simulink model "GFL_inverter2019a"  (R2019a)
settings: Solver=ode4  StartTime=0.0  StopTime=2  FixedStep=1e-6  RelTol=1e-3
values from neighbouring files (symbols this model uses):
  An1 = 0.01*funn    (= 0.3)    [dq_saopin_for_GFL_inverter.m]
  An2 = 0.03*funn    (= 0.9)    [dq_saopin_for_GFL_inverter.m]
  An3 = 0.05*funn    (= 1.5)    [dq_saopin_for_GFL_inverter.m]
  An4 = 0.07*funn    (= 2.1)    [dq_saopin_for_GFL_inverter.m]
  An5 = 0.09*funn    (= 2.7)    [dq_saopin_for_GFL_inverter.m]
  Ap1 = 0.01*funp    (= 0)    [dq_saopin_for_GFL_inverter.m]
  Ap2 = 0.03*funp    (= 0)    [dq_saopin_for_GFL_inverter.m]
  Ap3 = 0.05*funp    (= 0)    [dq_saopin_for_GFL_inverter.m]
  Ap4 = 0.07*funp    (= 0)    [dq_saopin_for_GFL_inverter.m]
  Ap5 = 0.09*funp    (= 0)    [dq_saopin_for_GFL_inverter.m]
  hp1 = hp0(n0)    [dq_saopin_for_GFL_inverter.m]
  hp2 = hp0(n0+hpn)    [dq_saopin_for_GFL_inverter.m]
  hp3 = hp0(n0+2*hpn)    [dq_saopin_for_GFL_inverter.m]
  hp4 = hp0(n0+3*hpn)    [dq_saopin_for_GFL_inverter.m]
  hp5 = hp0(n0+4*hpn)    [dq_saopin_for_GFL_inverter.m]
libraries: powerlib x27, powerlib_meascontrol x3, simulink x1
settings Model: Creator=18829  LastModifiedBy=wz
settings DataIOCC: ReturnWorkspaceOutputs=off
settings DebuggingCC: ArithmeticOperatorsInVariantConditions=warning
settings SFSimCC: SimUseLocalCustomCode=off
settings RTWCC: RTWUseLocalCustomCode=off
settings CodeAppCC: StateflowObjectComments=on
settings ConfigComp: CovBoundaryAbsTol=1.0e-5
settings SimscapeCC: SimscapeNormalizeSystem=off

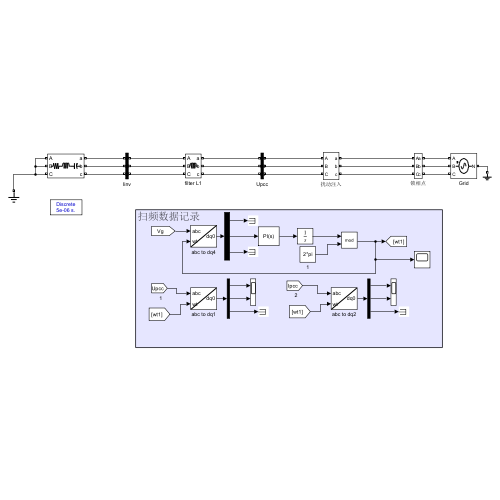
[thumbnail: Simulink's stored preview of the top-level diagram]
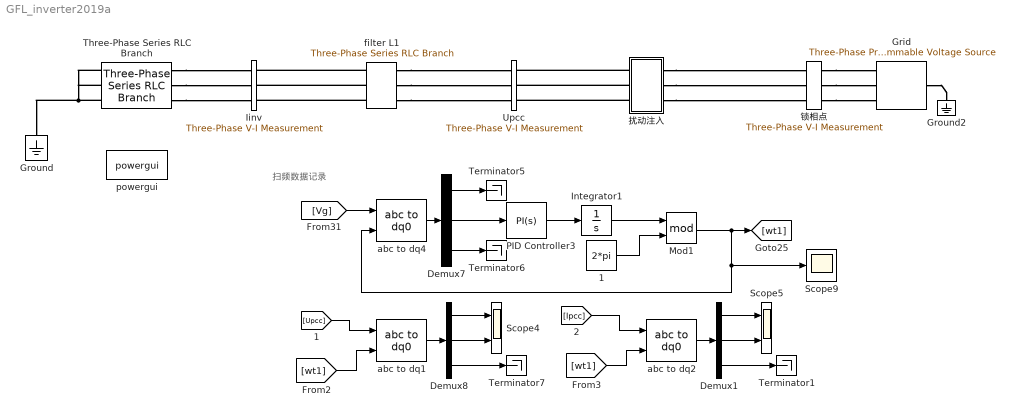
== system GFL_inverter2019a ==
  note: 扫频数据记录
  1 : Constant  Value=2*pi
  Demux1 : Demux  Outputs=3
  Demux7 : Demux  Outputs=3
  Demux8 : Demux  Outputs=3
  Grid : powerlib/Electrical Sources/Three-Phase Programmable Voltage Source  PositiveSequence=[380 0 50]  VariationEntity=None  VariationType=Table of time-amplitude pairs  VariationTypeAlt=Step  VariationStep=-3  VariationRate=10  VariationMagnitude=0.1  VariationFrequency=2  VariationTiming=[0.5 1.5]  VariationPhaseA=off  Amplitudes=[1 0.5 1]  TimeValues=[0 0.5 1]  HarmonicGeneration=off  HarmonicA=[7 0.1 0 0]  HarmonicB=[7 0.1 0 2]  Timing="[0.5  1]"  BusType=swing  Pref=0  Qref=0  Qmin=-inf  Qmax=inf
  Ground : powerlib/Elements/Ground  LConnTagsString=a
  Ground2 : powerlib/Elements/Ground  LConnTagsString=a
  Iinv : powerlib/Measurements/Three-Phase V-I Measurement  VoltageMeasurement=no  SetLabelV=off  LabelV=Uinv  Vpu=off  VpuLL=off  CurrentMeasurement=no  SetLabelI=off  LabelI=Iinv  Ipu=off  Pbase=100e6  Vbase=500e3  OutputType=Complex  PhasorSimulation=off  PSBequivalent=0
  Integrator1 : Integrator
  Mod1 : Math  Operator=mod  SaturateOnIntegerOverflow=on
  PID Controller3 : simulink/Continuous/PID Controller  Controller=PI  Form=Parallel  TimeDomain=Continuous-time  SampleTime=-1  IntegratorMethod=Forward Euler  ControllerParametersSource=internal  P=0.6935  I=74.885  D=0  N=100  UseFilter=on  TunerSelectOption=Transfer Function Based (PID Tuner App)  InitialConditionSource=internal  InitialConditionForIntegrator=100*pi  InitialConditionForFilter=0  DifferentiatorICPrevScaledInput=0  ExternalReset=none  TrackingMode=off  Kt=1  LimitOutput=off  UpperSaturationLimit=inf  LowerSaturationLimit=-inf  LinearizeAsGain=on  AntiWindupMode=none  Kb=1  POutMin=[]  POutMax=[]  IOutMin=[]  IOutMax=[]  DOutMin=[]  DOutMax=[]  NOutMin=[]  NOutMax=[]  SumOutMin=[]  SumOutMax=[]  SaturationOutMin=[]  SaturationOutMax=[]  PParamMin=[]  PParamMax=[]  IParamMin=[]  IParamMax=[]  DParamMin=[]  DParamMax=[]  NParamMin=[]  NParamMax=[]  KbParamMin=[]  KbParamMax=[]  KtParamMin=[]  KtParamMax=[]  KbOutMin=[]  KbOutMax=[]  KtOutMin=[]  KtOutMax=[]  IntegratorOutMin=[]  IntegratorOutMax=[]  FilterOutMin=[]  FilterOutMax=[]  SumI1OutMin=[]  SumI1OutMax=[]  SumI2OutMin=[]  SumI2OutMax=[]  SumI3OutMin=[]  SumI3OutMax=[]  SumI4OutMin=[]  SumI4OutMax=[]  SumDOutMin=[]  SumDOutMax=[]  DifferentiatorOutMin=[]  DifferentiatorOutMax=[]  FilterDiffOutCoefMin=[]  FilterDiffOutCoefMax=[]  ReciprocalOutMin=[]  ReciprocalOutMax=[]  SumDenOutMin=[]  SumDenOutMax=[]  SumNumOutMin=[]  SumNumOutMax=[]  DivideOutMin=[]  DivideOutMax=[]  IntegratorContinuousStateAttributes=''  IntegratorStateMustResolveToSignalObject=off  IntegratorRTWStateStorageClass=Auto  FilterContinuousStateAttributes=''  FilterStateMustResolveToSignalObject=off  FilterRTWStateStorageClass=Auto  ParallelPVariant=InternalParameters  IdealPVariant=Disabled  IVariant=InternalParameters  DVariant=Disabled  IntegratorVariant=Continuous  SatVariant=Disabled  AWVariant=Passthrough  PCopyVariant=Disabled  TRVariant=Disabled  FdbkBlocksVariant=Forward  IdealPFdbkVariant=Disabled  SatFdbkVariant=Disabled  DerivativeFilterVariant=Disabled  NVariant=Disabled  NCopyVariant=Disabled_SignalSpec  FilterICVariant=Disabled  IntegratorICVariant=InternalICs  ExternalResetVariant=Disabled  TRSumVariant=Passthrough  SumFdbkVariant=Disabled  SumVariant=Sum_PI
  Scope4 : Scope  NumInputPorts=2
  Scope5 : Scope  NumInputPorts=2
  Scope9 : Scope
  Terminator{1,5..7} (4 alike) : Terminator
  Three-Phase Series RLC Branch : powerlib/Elements/Three-Phase Series RLC Branch  LConnTagsString=A|B|C  RConnTagsString=A|B|C  BranchType=RLC  Resistance=1  Inductance=1e-3  Capacitance=0  Measurements=None
  Upcc : powerlib/Measurements/Three-Phase V-I Measurement  VoltageMeasurement=phase-to-ground  SetLabelV=on  LabelV=Upcc  Vpu=off  VpuLL=off  CurrentMeasurement=yes  SetLabelI=on  LabelI=Ipcc  Ipu=off  Pbase=100e6  Vbase=500e3  OutputType=Complex  PhasorSimulation=off  PSBequivalent=0
  abc to dq1 : powerlib_meascontrol/Transformations/abc to dq0  Alignment=90 degrees behind phase A axis
  abc to dq2 : powerlib_meascontrol/Transformations/abc to dq0  Alignment=90 degrees behind phase A axis
  abc to dq4 : powerlib_meascontrol/Transformations/abc to dq0  Alignment=90 degrees behind phase A axis
  filter L1 : powerlib/Elements/Three-Phase Series RLC Branch  LConnTagsString=A|B|C  RConnTagsString=A|B|C  BranchType=L  Resistance=0.01  Inductance=3e-3  Capacitance=1e-6  Measurements=None
  powergui : powerlib/powergui  Priority=1  SimulationMode=Discrete  SampleTime=5e-6  frequency=60  Iterations=50  frequencyindice=0  Pbase=100e6  ErrMax=1e-4  UnitsV=kV  UnitsW=MW  buscounter=0  FunctionMessages=off  echomessages=off  EnableUseOfTLC=off  CurrentSourceSwitches=off  DisableSnubberDevices=off  DisableRonSwitches=off  DisableVfSwitches=off  DisplayEquations=off  AutomaticDiscreteSolvers=off  SolverType=Tustin  Interpol=off  ExternalGateDelay=off  methode=off  Ts=0  x0status=blocks  SPID=off  SwTol=0  HookPort=off  NonlinearTolerance=1e-4  nMaxIteration=100  ContinueOnMaxIteration=off  RestoreLinks=warning  ResistiveCurrentMeasurement=off  Frange=[0:2:500]  Ylog=off  Xlog=on  ShowGrid=off  save=off  variable=ZData  structure=ScopeData1  ZoomFFT=off  StartTime=1.5  cycles=10  DisplayStyle=2  fundamental=50  FreqAxis=off  MaxFrequency=600  frequencyindicesteady=1  RmsSteady=1  display=off
  扰动注入 : Subsystem
  锁相点 : powerlib/Measurements/Three-Phase V-I Measurement  VoltageMeasurement=phase-to-ground  SetLabelV=on  LabelV=Vg  Vpu=off  VpuLL=off  CurrentMeasurement=no  SetLabelI=off  LabelI=Iabc  Ipu=off  Pbase=100e6  Vbase=500e3  OutputType=Complex  PhasorSimulation=off  PSBequivalent=0
  wires:
  1/1 -> Mod1/2
  PID Controller3/1 -> Integrator1/1
  Integrator1/1 -> Mod1/1
  Demux7/1 -> Terminator5/1
  Demux7/2 -> PID Controller3/1
  Demux7/3 -> Terminator6/1
  abc to dq4/1 -> Demux7/1
  [Vg] -> abc to dq4/1
  Mod1/1 -> [wt1], Scope9/1, abc to dq4/2
  [Upcc] -> abc to dq1/1
  [wt1] -> abc to dq1/2
  abc to dq1/1 -> Demux8/1
  Demux8/3 -> Terminator7/1
  Demux8/1 -> Scope4/1
  Demux8/2 -> Scope4/2
  Demux1/2 -> Scope5/2
  Demux1/1 -> Scope5/1
  Demux1/3 -> Terminator1/1
  abc to dq2/1 -> Demux1/1
  [wt1] -> abc to dq2/2
  [Ipcc] -> abc to dq2/1
  connections:
  Three-Phase Series RLC Branch/RConn1 -- Iinv/LConn1
  Grid/LConn1 -- Ground2/LConn1
  filter L1/LConn1 -- Iinv/RConn1
  Three-Phase Series RLC Branch/RConn3 -- Iinv/LConn3
  filter L1/LConn3 -- Iinv/RConn3
  Three-Phase Series RLC Branch/RConn2 -- Iinv/LConn2
  filter L1/LConn2 -- Iinv/RConn2
  锁相点/RConn1 -- Grid/RConn1
  锁相点/RConn2 -- Grid/RConn2
  锁相点/RConn3 -- Grid/RConn3
  filter L1/RConn1 -- Upcc/LConn1
  filter L1/RConn2 -- Upcc/LConn2
  filter L1/RConn3 -- Upcc/LConn3
  扰动注入/LConn1 -- Upcc/RConn1
  扰动注入/RConn1 -- 锁相点/LConn1
  扰动注入/LConn2 -- Upcc/RConn2
  扰动注入/RConn2 -- 锁相点/LConn2
  扰动注入/LConn3 -- Upcc/RConn3
  扰动注入/RConn3 -- 锁相点/LConn3
  Three-Phase Series RLC Branch/LConn3 -- Three-Phase Series RLC Branch/LConn1 -- Three-Phase Series RLC Branch/LConn2 -- Ground/LConn1

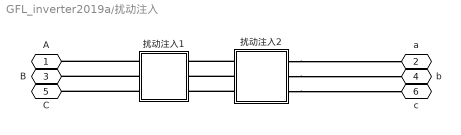
== system GFL_inverter2019a/扰动注入 ==
  扰动注入1 : Subsystem  mask{Ap1=Ap1, Ap2=Ap2, Ap3=Ap3, Ap4=Ap4, Ap5=Ap5, h1=hp1, h2=hp2, h3=hp3, h4=hp4, h5=hp5}
      mask DialogControl ParameterGroupVar Prompt: 参数
  扰动注入2 : Subsystem  mask{An1=An1, An2=An2, An3=An3, An4=An4, v5=An5, h1=hp1, h2=hp2, h3=hp3, h4=hp4, h5=hp5}
      mask prompts: v5 "An5"
      mask DialogControl ParameterGroupVar Prompt: 参数
  A : PMIOPort  Side=Left
  a : PMIOPort  Port=2  Side=Right
  B : PMIOPort  Port=3  Side=Left
  b : PMIOPort  Port=4  Side=Right
  C : PMIOPort  Port=5  Side=Left
  c : PMIOPort  Port=6  Side=Right
  connections:
  扰动注入2/RConn2 -- b/RConn1
  扰动注入2/LConn1 -- 扰动注入1/RConn1
  扰动注入1/LConn2 -- B/RConn1
  扰动注入2/LConn2 -- 扰动注入1/RConn2
  扰动注入2/LConn3 -- 扰动注入1/RConn3
  扰动注入2/RConn1 -- a/RConn1
  扰动注入1/LConn1 -- A/RConn1
  扰动注入1/LConn3 -- C/RConn1
  扰动注入2/RConn3 -- c/RConn1

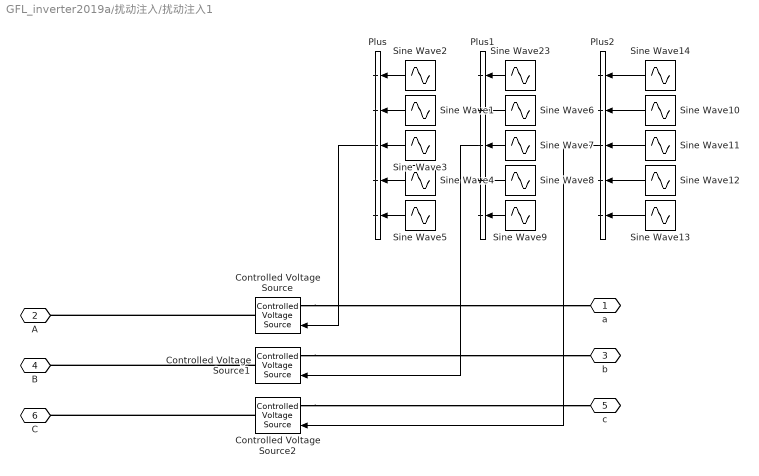
== system GFL_inverter2019a/扰动注入/扰动注入1 ==
  Controlled Voltage Source : powerlib/Electrical Sources/Controlled Voltage Source  Initialize=on  Source_Type=AC  Amplitude=0  Phase=0  Frequency=0  Measurements=None
  Controlled Voltage Source1 : powerlib/Electrical Sources/Controlled Voltage Source  Initialize=on  Source_Type=AC  Amplitude=0  Phase=0  Frequency=0  Measurements=None
  Controlled Voltage Source2 : powerlib/Electrical Sources/Controlled Voltage Source  Initialize=on  Source_Type=AC  Amplitude=0  Phase=0  Frequency=0  Measurements=None
  Plus : Sum  Inputs=+++++
  Plus1 : Sum  Inputs=+++++
  Plus2 : Sum  Inputs=+++++
  Sine Wave1 : Sin  Amplitude=Ap2  Frequency=2*pi*h2+2*pi*50  SampleTime=0
  Sine Wave10 : Sin  Amplitude=Ap2  Frequency=2*pi*h2+2*pi*50  Phase=+2*pi/3  SampleTime=0
  Sine Wave11 : Sin  Amplitude=Ap3  Frequency=2*pi*h3+2*pi*50  Phase=+2*pi/3  SampleTime=0
  Sine Wave12 : Sin  Amplitude=Ap4  Frequency=2*pi*h4+2*pi*50  Phase=+2*pi/3  SampleTime=0
  Sine Wave13 : Sin  Amplitude=Ap5  Frequency=2*pi*h5+2*pi*50  Phase=+2*pi/3  SampleTime=0
  Sine Wave14 : Sin  Amplitude=Ap1  Frequency=2*pi*h1+2*pi*50  Phase=+2*pi/3  SampleTime=0
  Sine Wave2 : Sin  Amplitude=Ap1  Frequency=2*pi*h1+2*pi*50  SampleTime=0
  Sine Wave23 : Sin  Amplitude=Ap1  Frequency=2*pi*h1+2*pi*50  Phase=-2*pi/3  SampleTime=0
  Sine Wave3 : Sin  Amplitude=Ap3  Frequency=2*pi*h3+2*pi*50  SampleTime=0
  Sine Wave4 : Sin  Amplitude=Ap4  Frequency=2*pi*h4+2*pi*50  SampleTime=0
  Sine Wave5 : Sin  Amplitude=Ap5  Frequency=2*pi*h5+2*pi*50  SampleTime=0
  Sine Wave6 : Sin  Amplitude=Ap2  Frequency=2*pi*h2+2*pi*50  Phase=-2*pi/3  SampleTime=0
  Sine Wave7 : Sin  Amplitude=Ap3  Frequency=2*pi*h3+2*pi*50  Phase=-2*pi/3  SampleTime=0
  Sine Wave8 : Sin  Amplitude=Ap4  Frequency=2*pi*h4+2*pi*50  Phase=-2*pi/3  SampleTime=0
  Sine Wave9 : Sin  Amplitude=Ap5  Frequency=2*pi*h5+2*pi*50  Phase=-2*pi/3  SampleTime=0
  a : PMIOPort  Side=Right
  A : PMIOPort  Port=2  Side=Left
  b : PMIOPort  Port=3  Side=Right
  B : PMIOPort  Port=4  Side=Left
  c : PMIOPort  Port=5  Side=Right
  C : PMIOPort  Port=6  Side=Left
  wires:
  Sine Wave2/1 -> Plus/1
  Sine Wave1/1 -> Plus/2
  Sine Wave3/1 -> Plus/3
  Sine Wave4/1 -> Plus/4
  Sine Wave5/1 -> Plus/5
  Plus/1 -> Controlled Voltage Source/1
  Plus1/1 -> Controlled Voltage Source1/1
  Sine Wave6/1 -> Plus1/2
  Sine Wave23/1 -> Plus1/1
  Sine Wave7/1 -> Plus1/3
  Sine Wave8/1 -> Plus1/4
  Sine Wave9/1 -> Plus1/5
  Sine Wave14/1 -> Plus2/1
  Sine Wave10/1 -> Plus2/2
  Sine Wave11/1 -> Plus2/3
  Sine Wave12/1 -> Plus2/4
  Sine Wave13/1 -> Plus2/5
  Plus2/1 -> Controlled Voltage Source2/1
  connections:
  Controlled Voltage Source1/LConn1 -- b/RConn1
  Controlled Voltage Source/LConn1 -- a/RConn1
  Controlled Voltage Source1/RConn1 -- B/RConn1
  Controlled Voltage Source/RConn1 -- A/RConn1
  Controlled Voltage Source2/LConn1 -- c/RConn1
  Controlled Voltage Source2/RConn1 -- C/RConn1

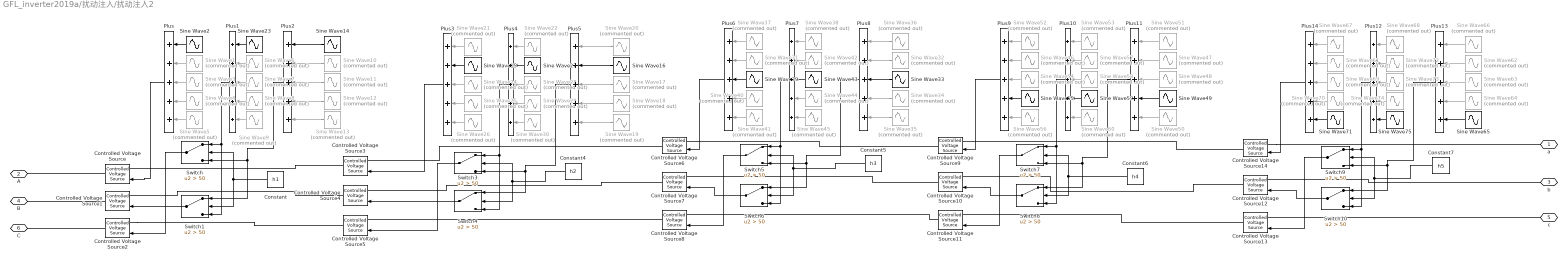
== system GFL_inverter2019a/扰动注入/扰动注入2 ==
  Constant : Constant  Value=h1
  Constant4 : Constant  Value=h2
  Constant5 : Constant  Value=h3
  Constant6 : Constant  Value=h4
  Constant7 : Constant  Value=h5
  Controlled Voltage Source{,1..14} (15 alike) : powerlib/Electrical Sources/Controlled Voltage Source  Initialize=on  Source_Type=AC  Amplitude=0  Phase=0  Frequency=0  Measurements=None
  Plus{,1..14} (15 alike) : Sum  Inputs=+++++
  Sine Wave{1,31,46,61} (4 alike) : Sin  Commented=on  Amplitude=An2  Frequency=abs(2*pi*h2-2*pi*50)  SampleTime=0
  Sine Wave{10,32,47,62} (4 alike) : Sin  Commented=on  Amplitude=An2  Frequency=abs(2*pi*h2-2*pi*50)  Phase=+2*pi/3  SampleTime=0
  Sine Wave{11,17,48,63} (4 alike) : Sin  Commented=on  Amplitude=An3  Frequency=abs(2*pi*h3-2*pi*50)  Phase=+2*pi/3  SampleTime=0
  Sine Wave12 : Sin  Commented=on  Amplitude=An4  Frequency=abs(2*pi*h4-2*pi*50)  Phase=+2*pi/3  SampleTime=0
  Sine Wave13 : Sin  Commented=on  Amplitude=An5  Frequency=abs(2*pi*h5-2*pi*50)  Phase=+2*pi/3  SampleTime=0
  Sine Wave14 : Sin  Amplitude=An1  Frequency=abs(2*pi*h1-2*pi*50)  Phase=+2*pi/3  SampleTime=0
  Sine Wave15 : Sin  Amplitude=An2  Frequency=abs(2*pi*h2-2*pi*50)  SampleTime=0
  Sine Wave16 : Sin  Amplitude=An2  Frequency=abs(2*pi*h2-2*pi*50)  Phase=+2*pi/3  SampleTime=0
  Sine Wave18 : Sin  Commented=on  Amplitude=An4  Frequency=2*pi*h4  Phase=+2*pi/3  SampleTime=0
  Sine Wave19 : Sin  Commented=on  Amplitude=An5  Frequency=2*pi*h5  Phase=+2*pi/3  SampleTime=0
  Sine Wave2 : Sin  Amplitude=An1  Frequency=abs(2*pi*h1-2*pi*50)  SampleTime=0
  Sine Wave{20,36,51,66} (4 alike) : Sin  Commented=on  Amplitude=An1  Frequency=abs(2*pi*h1-2*pi*50)  Phase=+2*pi/3  SampleTime=0
  Sine Wave{21,37,52,67} (4 alike) : Sin  Commented=on  Amplitude=An1  Frequency=abs(2*pi*h1-2*pi*50)  SampleTime=0
  Sine Wave{22,38,53,68} (4 alike) : Sin  Commented=on  Amplitude=An1  Frequency=abs(2*pi*h1-2*pi*50)  Phase=-2*pi/3  SampleTime=0
  Sine Wave23 : Sin  Amplitude=An1  Frequency=abs(2*pi*h1-2*pi*50)  Phase=-2*pi/3  SampleTime=0
  Sine Wave{3,24,54,69} (4 alike) : Sin  Commented=on  Amplitude=An3  Frequency=abs(2*pi*h3-2*pi*50)  SampleTime=0
  Sine Wave25 : Sin  Commented=on  Amplitude=An4  Frequency=2*pi*h4  SampleTime=0
  Sine Wave26 : Sin  Commented=on  Amplitude=An5  Frequency=2*pi*h5  SampleTime=0
  Sine Wave27 : Sin  Amplitude=An2  Frequency=abs(2*pi*h2-2*pi*50)  Phase=-2*pi/3  SampleTime=0
  Sine Wave{7,28,58,73} (4 alike) : Sin  Commented=on  Amplitude=An3  Frequency=abs(2*pi*h3-2*pi*50)  Phase=-2*pi/3  SampleTime=0
  Sine Wave29 : Sin  Commented=on  Amplitude=An4  Frequency=2*pi*h4  Phase=-2*pi/3  SampleTime=0
  Sine Wave30 : Sin  Commented=on  Amplitude=An5  Frequency=2*pi*h5  Phase=-2*pi/3  SampleTime=0
  Sine Wave33 : Sin  Amplitude=An3  Frequency=abs(2*pi*h3-2*pi*50)  Phase=+2*pi/3  SampleTime=0
  Sine Wave34 : Sin  Commented=on  Amplitude=An4  Frequency=2*pi*h4  Phase=+2*pi/3  SampleTime=0
  Sine Wave35 : Sin  Commented=on  Amplitude=An5  Frequency=2*pi*h5  Phase=+2*pi/3  SampleTime=0
  Sine Wave39 : Sin  Amplitude=An3  Frequency=abs(2*pi*h3-2*pi*50)  SampleTime=0
  Sine Wave4 : Sin  Commented=on  Amplitude=An4  Frequency=abs(2*pi*h4-2*pi*50)  SampleTime=0
  Sine Wave40 : Sin  Commented=on  Amplitude=An4  Frequency=2*pi*h4  SampleTime=0
  Sine Wave41 : Sin  Commented=on  Amplitude=An5  Frequency=2*pi*h5  SampleTime=0
  Sine Wave{6,42,57,72} (4 alike) : Sin  Commented=on  Amplitude=An2  Frequency=abs(2*pi*h2-2*pi*50)  Phase=-2*pi/3  SampleTime=0
  Sine Wave43 : Sin  Amplitude=An3  Frequency=abs(2*pi*h3-2*pi*50)  Phase=-2*pi/3  SampleTime=0
  Sine Wave44 : Sin  Commented=on  Amplitude=An4  Frequency=2*pi*h4  Phase=-2*pi/3  SampleTime=0
  Sine Wave45 : Sin  Commented=on  Amplitude=An5  Frequency=2*pi*h5  Phase=-2*pi/3  SampleTime=0
  Sine Wave49 : Sin  Amplitude=An4  Frequency=abs(2*pi*h4-2*pi*50)  Phase=+2*pi/3  SampleTime=0
  Sine Wave5 : Sin  Commented=on  Amplitude=An5  Frequency=abs(2*pi*h5-2*pi*50)  SampleTime=0
  Sine Wave50 : Sin  Commented=on  Amplitude=An5  Frequency=2*pi*h5  Phase=+2*pi/3  SampleTime=0
  Sine Wave55 : Sin  Amplitude=An4  Frequency=abs(2*pi*h4-2*pi*50)  SampleTime=0
  Sine Wave56 : Sin  Commented=on  Amplitude=An5  Frequency=2*pi*h5  SampleTime=0
  Sine Wave59 : Sin  Amplitude=An4  Frequency=abs(2*pi*h4-2*pi*50)  Phase=-2*pi/3  SampleTime=0
  Sine Wave60 : Sin  Commented=on  Amplitude=An5  Frequency=2*pi*h5  Phase=-2*pi/3  SampleTime=0
  Sine Wave64 : Sin  Commented=on  Amplitude=An4  Frequency=abs(2*pi*h4-2*pi*50)  Phase=+2*pi/3  SampleTime=0
  Sine Wave65 : Sin  Amplitude=An5  Frequency=abs(2*pi*h5-2*pi*50)  Phase=+2*pi/3  SampleTime=0
  Sine Wave70 : Sin  Commented=on  Amplitude=An4  Frequency=abs(2*pi*h4-2*pi*50)  SampleTime=0
  Sine Wave71 : Sin  Amplitude=An5  Frequency=abs(2*pi*h5-2*pi*50)  SampleTime=0
  Sine Wave74 : Sin  Commented=on  Amplitude=An4  Frequency=abs(2*pi*h4-2*pi*50)  Phase=-2*pi/3  SampleTime=0
  Sine Wave75 : Sin  Amplitude=An5  Frequency=abs(2*pi*h5-2*pi*50)  Phase=-2*pi/3  SampleTime=0
  Sine Wave8 : Sin  Commented=on  Amplitude=An4  Frequency=abs(2*pi*h4-2*pi*50)  Phase=-2*pi/3  SampleTime=0
  Sine Wave9 : Sin  Commented=on  Amplitude=An5  Frequency=abs(2*pi*h5-2*pi*50)  Phase=-2*pi/3  SampleTime=0
  Switch{,1,3..10} (10 alike) : Switch  Criteria=u2 > Threshold  Threshold=50
  a : PMIOPort  Side=Right
  A : PMIOPort  Port=2  Side=Left
  b : PMIOPort  Port=3  Side=Right
  B : PMIOPort  Port=4  Side=Left
  c : PMIOPort  Port=5  Side=Right
  C : PMIOPort  Port=6  Side=Left
  wires:
  Sine Wave13/1 -> Plus2/5
  Sine Wave12/1 -> Plus2/4
  Sine Wave11/1 -> Plus2/3
  Sine Wave10/1 -> Plus2/2
  Sine Wave14/1 -> Plus2/1
  Sine Wave9/1 -> Plus1/5
  Sine Wave8/1 -> Plus1/4
  Sine Wave7/1 -> Plus1/3
  Sine Wave23/1 -> Plus1/1
  Sine Wave6/1 -> Plus1/2
  Plus/1 -> Controlled Voltage Source/1
  Sine Wave5/1 -> Plus/5
  Sine Wave4/1 -> Plus/4
  Sine Wave3/1 -> Plus/3
  Sine Wave1/1 -> Plus/2
  Sine Wave2/1 -> Plus/1
  Plus2/1 -> Switch1/1, Switch/3
  Plus1/1 -> Switch/1, Switch1/3
  Constant/1 -> Switch1/2, Switch/2
  Switch/1 -> Controlled Voltage Source2/1
  Switch1/1 -> Controlled Voltage Source1/1
  Switch4/1 -> Controlled Voltage Source4/1
  Switch3/1 -> Controlled Voltage Source5/1
  Constant4/1 -> Switch4/2, Switch3/2
  Plus4/1 -> Switch4/3, Switch3/1
  Plus5/1 -> Switch3/3, Switch4/1
  Sine Wave21/1 -> Plus3/1
  Sine Wave15/1 -> Plus3/2
  Sine Wave24/1 -> Plus3/3
  Sine Wave25/1 -> Plus3/4
  Sine Wave26/1 -> Plus3/5
  Plus3/1 -> Controlled Voltage Source3/1
  Sine Wave27/1 -> Plus4/2
  Sine Wave22/1 -> Plus4/1
  Sine Wave28/1 -> Plus4/3
  Sine Wave29/1 -> Plus4/4
  Sine Wave30/1 -> Plus4/5
  Sine Wave20/1 -> Plus5/1
  Sine Wave16/1 -> Plus5/2
  Sine Wave17/1 -> Plus5/3
  Sine Wave18/1 -> Plus5/4
  Sine Wave19/1 -> Plus5/5
  Sine Wave35/1 -> Plus8/5
  Sine Wave34/1 -> Plus8/4
  Sine Wave33/1 -> Plus8/3
  Sine Wave32/1 -> Plus8/2
  Sine Wave36/1 -> Plus8/1
  Sine Wave45/1 -> Plus7/5
  Sine Wave44/1 -> Plus7/4
  Sine Wave43/1 -> Plus7/3
  Sine Wave38/1 -> Plus7/1
  Sine Wave42/1 -> Plus7/2
  Plus6/1 -> Controlled Voltage Source6/1
  Sine Wave41/1 -> Plus6/5
  Sine Wave40/1 -> Plus6/4
  Sine Wave39/1 -> Plus6/3
  Sine Wave31/1 -> Plus6/2
  Sine Wave37/1 -> Plus6/1
  Plus8/1 -> Switch6/1, Switch5/3
  Plus7/1 -> Switch5/1, Switch6/3
  Constant5/1 -> Switch6/2, Switch5/2
  Switch5/1 -> Controlled Voltage Source8/1
  Switch6/1 -> Controlled Voltage Source7/1
  Switch8/1 -> Controlled Voltage Source10/1
  Switch7/1 -> Controlled Voltage Source11/1
  Constant6/1 -> Switch7/2, Switch8/2
  Plus10/1 -> Switch8/3, Switch7/1
  Plus11/1 -> Switch7/3, Switch8/1
  Sine Wave52/1 -> Plus9/1
  Sine Wave46/1 -> Plus9/2
  Sine Wave54/1 -> Plus9/3
  Sine Wave55/1 -> Plus9/4
  Sine Wave56/1 -> Plus9/5
  Plus9/1 -> Controlled Voltage Source9/1
  Sine Wave57/1 -> Plus10/2
  Sine Wave53/1 -> Plus10/1
  Sine Wave58/1 -> Plus10/3
  Sine Wave59/1 -> Plus10/4
  Sine Wave60/1 -> Plus10/5
  Sine Wave51/1 -> Plus11/1
  Sine Wave47/1 -> Plus11/2
  Sine Wave48/1 -> Plus11/3
  Sine Wave49/1 -> Plus11/4
  Sine Wave50/1 -> Plus11/5
  Sine Wave65/1 -> Plus13/5
  Sine Wave64/1 -> Plus13/4
  Sine Wave63/1 -> Plus13/3
  Sine Wave62/1 -> Plus13/2
  Sine Wave66/1 -> Plus13/1
  Sine Wave75/1 -> Plus12/5
  Sine Wave74/1 -> Plus12/4
  Sine Wave73/1 -> Plus12/3
  Sine Wave68/1 -> Plus12/1
  Sine Wave72/1 -> Plus12/2
  Plus14/1 -> Controlled Voltage Source14/1
  Sine Wave71/1 -> Plus14/5
  Sine Wave70/1 -> Plus14/4
  Sine Wave69/1 -> Plus14/3
  Sine Wave61/1 -> Plus14/2
  Sine Wave67/1 -> Plus14/1
  Plus13/1 -> Switch10/1, Switch9/3
  Plus12/1 -> Switch9/1, Switch10/3
  Constant7/1 -> Switch10/2, Switch9/2
  Switch9/1 -> Controlled Voltage Source13/1
  Switch10/1 -> Controlled Voltage Source12/1
  connections:
  Controlled Voltage Source2/RConn1 -- C/RConn1
  Controlled Voltage Source/RConn1 -- A/RConn1
  Controlled Voltage Source1/RConn1 -- B/RConn1
  Controlled Voltage Source3/RConn1 -- Controlled Voltage Source/LConn1
  Controlled Voltage Source4/RConn1 -- Controlled Voltage Source1/LConn1
  Controlled Voltage Source2/LConn1 -- Controlled Voltage Source5/RConn1
  Controlled Voltage Source6/RConn1 -- Controlled Voltage Source3/LConn1
  Controlled Voltage Source7/RConn1 -- Controlled Voltage Source4/LConn1
  Controlled Voltage Source8/RConn1 -- Controlled Voltage Source5/LConn1
  Controlled Voltage Source9/RConn1 -- Controlled Voltage Source6/LConn1
  Controlled Voltage Source10/RConn1 -- Controlled Voltage Source7/LConn1
  Controlled Voltage Source11/RConn1 -- Controlled Voltage Source8/LConn1
  Controlled Voltage Source14/RConn1 -- Controlled Voltage Source9/LConn1
  Controlled Voltage Source12/RConn1 -- Controlled Voltage Source10/LConn1
  Controlled Voltage Source13/RConn1 -- Controlled Voltage Source11/LConn1
  Controlled Voltage Source14/LConn1 -- a/RConn1
  b/RConn1 -- Controlled Voltage Source12/LConn1
  c/RConn1 -- Controlled Voltage Source13/LConn1
